simulink model "PMLSM_MIL_ControlCore_Sim"  (R2026a)
settings: Solver=FixedStepDiscrete  StopTime=MIL_StopTime_s  FixedStep=MIL_Ts_s
InitFcn:
  | init_PMLSM_control_params; init_PMLSM_plant_params; init_PMLSM_mil_test_params;
values from neighbouring files (symbols this model uses):
  Inverter_DeadTime_Mode = 0    [init_PMLSM_mil_test_params.m]
  MIL_Current_Control_Ts_s = 1e-4    (= 0.0001)    [init_PMLSM_mil_test_params.m]
  MIL_EnableTime_s = 0.1    [init_PMLSM_mil_test_params.m]
  MIL_Fault_Start_s = 2.0    (= 2)    [init_PMLSM_mil_test_params.m]
  MIL_Fault_Test_Case = 0    [init_PMLSM_mil_test_params.m]
  MIL_InitDoneDelay_s = 1    [init_PMLSM_mil_test_params.m]
  MIL_Mode = 1    [init_PMLSM_mil_test_params.m]
  MIL_PWM_Delay_Substep_s = MIL_Ts_s    (= 0.0001)    [init_PMLSM_mil_test_params.m]
  MIL_PWM_Update_Delay_Accurate_Enable = 0    [init_PMLSM_mil_test_params.m]
  MIL_PWM_Update_Delay_Mode = 1    [init_PMLSM_mil_test_params.m]
  MIL_StaticCurrentStepTest_Enable = 1    [init_PMLSM_mil_test_params.m]
  MIL_Ts_s = 1e-4    (= 0.0001)    [init_PMLSM_mil_test_params.m]
  Plant_Input_Mode = 2    [init_PMLSM_mil_test_params.m]
  PMLSM_Bv_N_per_mps = 0    [init_PMLSM_ThreeLoop_Simple.m]    (also in init_PMLSM_plant_params.m)
  PMLSM_deadtime_current_eps_A = 1e-4    (= 0.0001)    [init_PMLSM_ThreeLoop_Simple.m]    (also in init_PMLSM_plant_params.m)
  PMLSM_deadtime_ratio = PMLSM_deadtime_s/Ts    (= 0.01)    [init_PMLSM_ThreeLoop_Simple.m]    (also in init_PMLSM_plant_params.m)
  PMLSM_Fc_N = 0    [init_PMLSM_ThreeLoop_Simple.m]    (also in init_PMLSM_plant_params.m)
  PMLSM_grating_resolution_mm = 0.0001    [init_PMLSM_plant_params.m]
  PMLSM_Kf_peak_N_per_Apeak = 31.4/sqrt(2)    [init_PMLSM_ThreeLoop_Simple.m]    (also in init_PMLSM_plant_params.m = PMLSM_Kf_rms_N_per_Arms/sqrt(2))
  PMLSM_Ld_H = Ld    (= 0.001745)    [PMSLM_Init_Params_MBDL4.m]    (also in init_PMLSM_ThreeLoop_Simple.m; init_PMLSM_plant_params.m)
  PMLSM_Lq_H = Lq    (= 0.001745)    [PMSLM_Init_Params_MBDL4.m]    (also in init_PMLSM_ThreeLoop_Simple.m; init_PMLSM_plant_params.m)
  PMLSM_M_kg = 0.91    [init_PMLSM_ThreeLoop_Simple.m]    (also in init_PMLSM_plant_params.m)
  PMLSM_psi_f_Wb = flux    (= 0.141)    [PMSLM_Init_Params_MBDL4.m]    (also in init_PMLSM_ThreeLoop_Simple.m; init_PMLSM_plant_params.m)
  PMLSM_pwm_period_counts = CPU_Clock*Ts/2    (= 10000)    [init_PMLSM_ThreeLoop_Simple.m]    (also in init_PMLSM_plant_params.m = 7500)
  PMLSM_Rs_ohm = Rs    (= 2.37)    [PMSLM_Init_Params_MBDL4.m]    (also in init_PMLSM_ThreeLoop_Simple.m; init_PMLSM_plant_params.m)
  PMLSM_sensor_delay_samples = 50    [init_PMLSM_plant_params.m]
  PMLSM_tau_NN_m = 0.06    [init_PMLSM_ThreeLoop_Simple.m]    (also in init_PMLSM_plant_params.m)
  PMLSM_theta_offset_rad = 0    [init_PMLSM_ThreeLoop_Simple.m]    (also in init_PMLSM_plant_params.m)
  PMLSM_Ts_s = Ts/2    (= 5e-05)    [init_PMLSM_ThreeLoop_Simple.m]    (also in init_PMLSM_plant_params.m = 0.0001)
  PMLSM_v_eps_mps = 1e-3    (= 0.001)    [init_PMLSM_ThreeLoop_Simple.m]    (also in init_PMLSM_plant_params.m)
  Ts_ACR = 1e-4    (= 0.0001)    [PMSLM_Init_Params_MBDL4.m]    (also in init_PMLSM_ThreeLoop_Simple.m)
undefined symbols (not defined in the file or in its folder): DiscIntNeverNeededParam
settings Model: Creator=lww  LastModifiedBy=lww

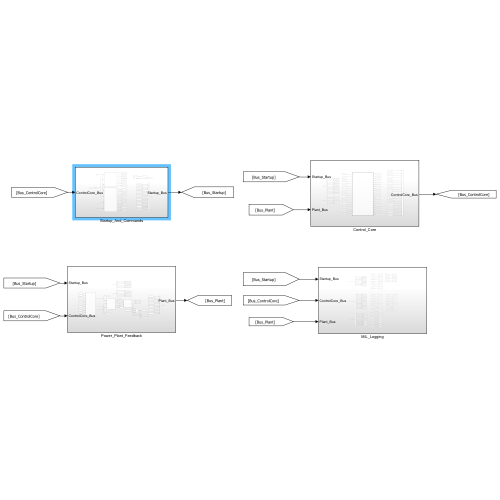
[thumbnail: Simulink's stored preview of the top-level diagram]
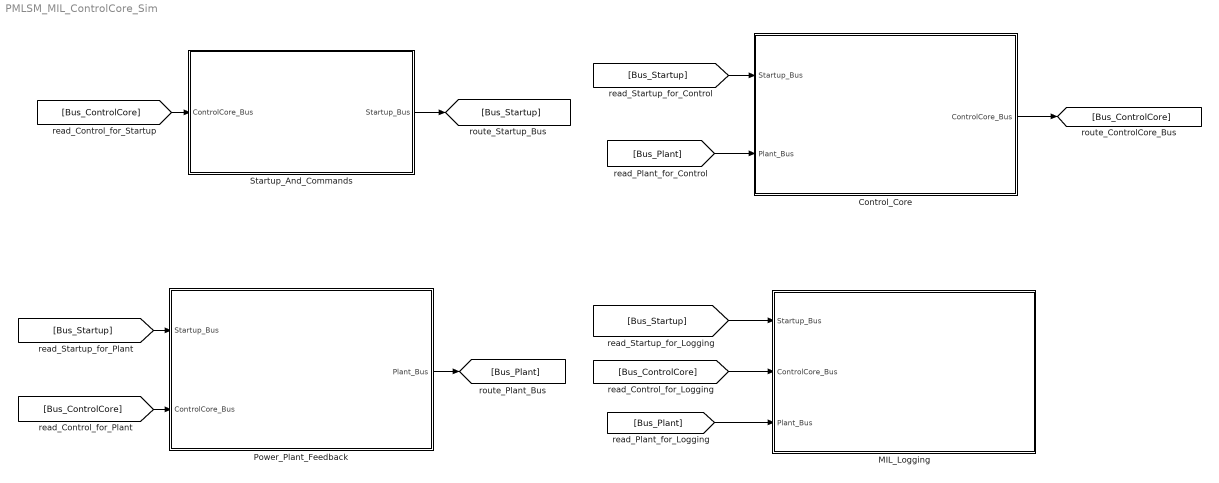
== system PMLSM_MIL_ControlCore_Sim ==
  Control_Core : Subsystem
  MIL_Logging : Subsystem
  Power_Plant_Feedback : Subsystem
  Startup_And_Commands : Subsystem
  wires:
  Startup_And_Commands/1(Startup_Bus) -> [Bus_Startup]
  [Bus_Startup] -> Control_Core/1(Startup_Bus)
  [Bus_Startup] -> Power_Plant_Feedback/1(Startup_Bus)
  [Bus_Startup] -> MIL_Logging/1(Startup_Bus)
  Control_Core/1(ControlCore_Bus) -> [Bus_ControlCore]
  [Bus_ControlCore] -> Startup_And_Commands/1(ControlCore_Bus)
  [Bus_ControlCore] -> Power_Plant_Feedback/2(ControlCore_Bus)
  [Bus_ControlCore] -> MIL_Logging/2(ControlCore_Bus)
  Power_Plant_Feedback/1(Plant_Bus) -> [Bus_Plant]
  [Bus_Plant] -> Control_Core/2(Plant_Bus)
  [Bus_Plant] -> MIL_Logging/3(Plant_Bus)

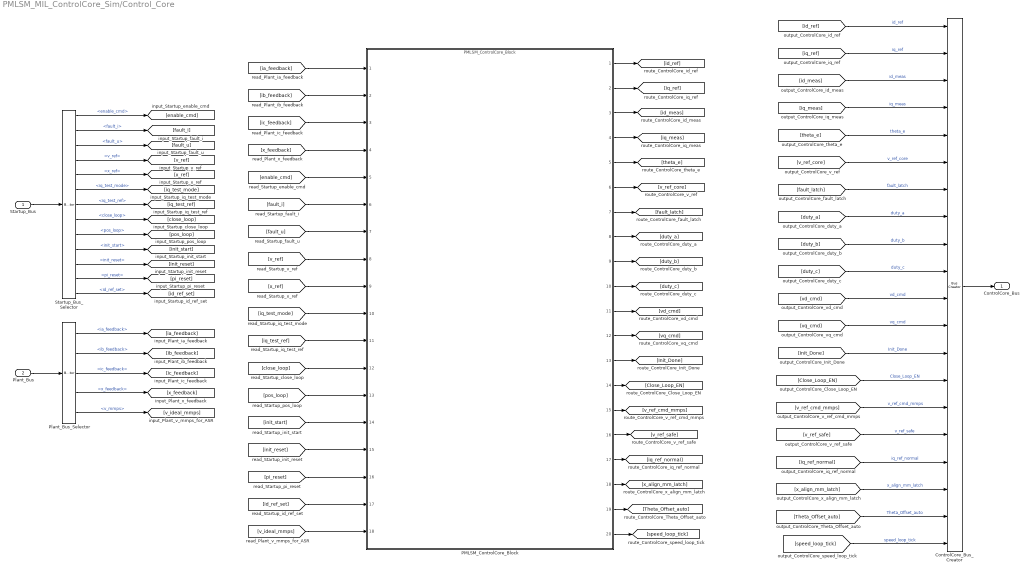
== system PMLSM_MIL_ControlCore_Sim/Control_Core ==
  Startup_Bus : Inport
  Plant_Bus : Inport  Port=2
  ControlCore_Bus_Creator : BusCreator  Inputs=20
  PMLSM_ControlCore_Block : ModelReference  ModelNameDialog=PMLSM_ControlCore_Block  SimulationMode=Normal  ModelReferenceVersion=6.250
  Plant_Bus_Selector : BusSelector  OutputSignals=ia_feedback,ib_feedback,ic_feedback,x_feedback,v_mmps
  Startup_Bus_Selector : BusSelector  OutputSignals=enable_cmd,fault_i,fault_u,v_ref,x_ref,iq_test_mode,iq_test_ref,close_loop,pos_loop,init_start,init_reset,pi_reset,id_ref_set
  ControlCore_Bus : Outport
  wires:
  Startup_Bus/1 -> Startup_Bus_Selector/1
  Startup_Bus_Selector/1 -> [enable_cmd]  "<enable_cmd>"
  Startup_Bus_Selector/2 -> [fault_i]  "<fault_i>"
  Startup_Bus_Selector/3 -> [fault_u]  "<fault_u>"
  Startup_Bus_Selector/4 -> [v_ref]  "<v_ref>"
  Startup_Bus_Selector/5 -> [x_ref]  "<x_ref>"
  Startup_Bus_Selector/6 -> [iq_test_mode]  "<iq_test_mode>"
  Startup_Bus_Selector/7 -> [iq_test_ref]  "<iq_test_ref>"
  Startup_Bus_Selector/8 -> [close_loop]  "<close_loop>"
  Startup_Bus_Selector/9 -> [pos_loop]  "<pos_loop>"
  Startup_Bus_Selector/10 -> [init_start]  "<init_start>"
  Startup_Bus_Selector/11 -> [init_reset]  "<init_reset>"
  Startup_Bus_Selector/12 -> [pi_reset]  "<pi_reset>"
  Startup_Bus_Selector/13 -> [id_ref_set]  "<id_ref_set>"
  Plant_Bus/1 -> Plant_Bus_Selector/1
  Plant_Bus_Selector/1 -> [ia_feedback]  "<ia_feedback>"
  Plant_Bus_Selector/2 -> [ib_feedback]  "<ib_feedback>"
  Plant_Bus_Selector/3 -> [ic_feedback]  "<ic_feedback>"
  Plant_Bus_Selector/4 -> [x_feedback]  "<x_feedback>"
  [ia_feedback] -> PMLSM_ControlCore_Block/1
  [ib_feedback] -> PMLSM_ControlCore_Block/2
  [ic_feedback] -> PMLSM_ControlCore_Block/3
  [x_feedback] -> PMLSM_ControlCore_Block/4
  [enable_cmd] -> PMLSM_ControlCore_Block/5
  [fault_i] -> PMLSM_ControlCore_Block/6
  [fault_u] -> PMLSM_ControlCore_Block/7
  [v_ref] -> PMLSM_ControlCore_Block/8
  [x_ref] -> PMLSM_ControlCore_Block/9
  [iq_test_mode] -> PMLSM_ControlCore_Block/10
  [iq_test_ref] -> PMLSM_ControlCore_Block/11
  [close_loop] -> PMLSM_ControlCore_Block/12
  [pos_loop] -> PMLSM_ControlCore_Block/13
  [init_start] -> PMLSM_ControlCore_Block/14
  [init_reset] -> PMLSM_ControlCore_Block/15
  [pi_reset] -> PMLSM_ControlCore_Block/16
  [id_ref_set] -> PMLSM_ControlCore_Block/17
  PMLSM_ControlCore_Block/1 -> [id_ref]
  PMLSM_ControlCore_Block/2 -> [iq_ref]
  PMLSM_ControlCore_Block/3 -> [id_meas]
  PMLSM_ControlCore_Block/4 -> [iq_meas]
  PMLSM_ControlCore_Block/5 -> [theta_e]
  PMLSM_ControlCore_Block/6 -> [v_ref_core]
  PMLSM_ControlCore_Block/7 -> [fault_latch]
  PMLSM_ControlCore_Block/8 -> [duty_a]
  PMLSM_ControlCore_Block/9 -> [duty_b]
  PMLSM_ControlCore_Block/10 -> [duty_c]
  PMLSM_ControlCore_Block/11 -> [vd_cmd]
  PMLSM_ControlCore_Block/12 -> [vq_cmd]
  PMLSM_ControlCore_Block/13 -> [Init_Done]
  PMLSM_ControlCore_Block/14 -> [Close_Loop_EN]
  PMLSM_ControlCore_Block/15 -> [v_ref_cmd_mmps]
  PMLSM_ControlCore_Block/16 -> [v_ref_safe]
  PMLSM_ControlCore_Block/17 -> [iq_ref_normal]
  PMLSM_ControlCore_Block/18 -> [x_align_mm_latch]
  PMLSM_ControlCore_Block/19 -> [Theta_Offset_auto]
  [id_ref] -> ControlCore_Bus_Creator/1  "id_ref"
  [iq_ref] -> ControlCore_Bus_Creator/2  "iq_ref"
  [id_meas] -> ControlCore_Bus_Creator/3  "id_meas"
  [iq_meas] -> ControlCore_Bus_Creator/4  "iq_meas"
  [theta_e] -> ControlCore_Bus_Creator/5  "theta_e"
  [v_ref_core] -> ControlCore_Bus_Creator/6  "v_ref_core"
  [fault_latch] -> ControlCore_Bus_Creator/7  "fault_latch"
  [duty_a] -> ControlCore_Bus_Creator/8  "duty_a"
  [duty_b] -> ControlCore_Bus_Creator/9  "duty_b"
  [duty_c] -> ControlCore_Bus_Creator/10  "duty_c"
  [vd_cmd] -> ControlCore_Bus_Creator/11  "vd_cmd"
  [vq_cmd] -> ControlCore_Bus_Creator/12  "vq_cmd"
  [Init_Done] -> ControlCore_Bus_Creator/13  "Init_Done"
  [Close_Loop_EN] -> ControlCore_Bus_Creator/14  "Close_Loop_EN"
  [v_ref_cmd_mmps] -> ControlCore_Bus_Creator/15  "v_ref_cmd_mmps"
  [v_ref_safe] -> ControlCore_Bus_Creator/16  "v_ref_safe"
  [iq_ref_normal] -> ControlCore_Bus_Creator/17  "iq_ref_normal"
  [x_align_mm_latch] -> ControlCore_Bus_Creator/18  "x_align_mm_latch"
  [Theta_Offset_auto] -> ControlCore_Bus_Creator/19  "Theta_Offset_auto"
  ControlCore_Bus_Creator/1 -> ControlCore_Bus/1
  Plant_Bus_Selector/5 -> [v_ideal_mmps]  "<v_mmps>"
  [v_ideal_mmps] -> PMLSM_ControlCore_Block/18
  PMLSM_ControlCore_Block/20 -> [speed_loop_tick]
  [speed_loop_tick] -> ControlCore_Bus_Creator/20  "speed_loop_tick"

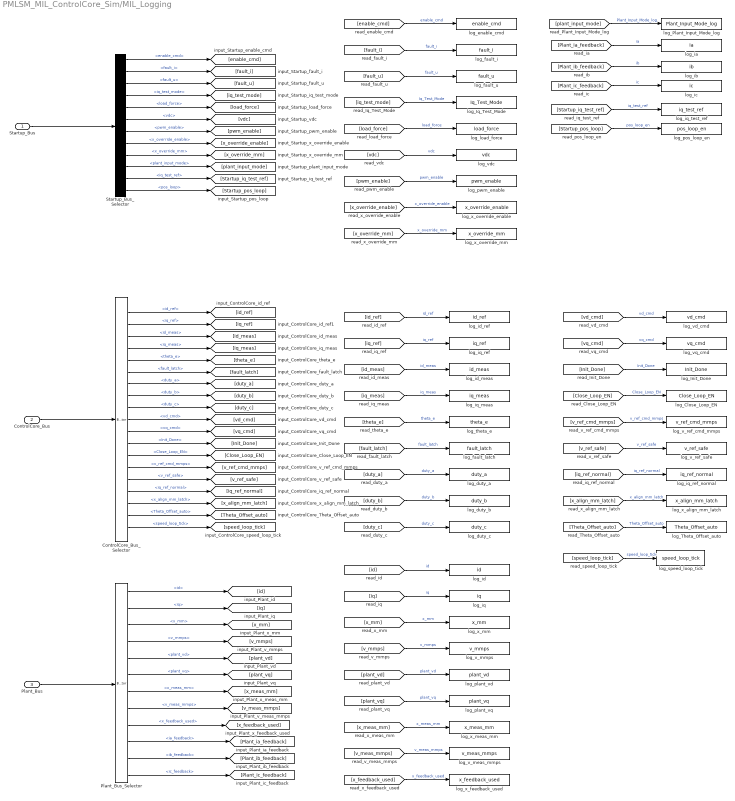
== system PMLSM_MIL_ControlCore_Sim/MIL_Logging ==
  Startup_Bus : Inport
  ControlCore_Bus : Inport  Port=2
  Plant_Bus : Inport  Port=3
  ControlCore_Bus_Selector : BusSelector  OutputSignals=id_ref,iq_ref,id_meas,iq_meas,theta_e,fault_latch,duty_a,duty_b,duty_c,vd_cmd,vq_cmd,Init_Done,Close_Loop_EN,v_ref_cmd_mmps,v_ref_safe,iq_ref_normal,x_align_mm_latch,Theta_Offset_auto,speed_loop_tick
  Plant_Bus_Selector : BusSelector  OutputSignals=id,iq,x_mm,v_mmps,plant_vd,plant_vq,x_meas_mm,v_meas_mmps,x_feedback_used,ia_feedback,ib_feedback,ic_feedback
  Startup_Bus_Selector : BusSelector  OutputSignals=enable_cmd,fault_i,fault_u,iq_test_mode,load_force,vdc,pwm_enable,x_override_enable,x_override_mm,plant_input_mode,iq_test_ref,pos_loop
  log_Close_Loop_EN : ToWorkspace  VariableName=Close_Loop_EN  SaveFormat=Timeseries  SampleTime=-1
  log_Init_Done : ToWorkspace  VariableName=Init_Done  SaveFormat=Timeseries  SampleTime=-1
  log_Iq_Test_Mode : ToWorkspace  VariableName=Iq_Test_Mode  SaveFormat=Timeseries  SampleTime=-1
  log_Plant_Input_Mode_log : ToWorkspace  VariableName=Plant_Input_Mode_log  SaveFormat=Timeseries  SampleTime=-1
  log_Theta_Offset_auto : ToWorkspace  VariableName=Theta_Offset_auto  SaveFormat=Timeseries  SampleTime=-1
  log_duty_a : ToWorkspace  VariableName=duty_a  SaveFormat=Timeseries  SampleTime=-1
  log_duty_b : ToWorkspace  VariableName=duty_b  SaveFormat=Timeseries  SampleTime=-1
  log_duty_c : ToWorkspace  VariableName=duty_c  SaveFormat=Timeseries  SampleTime=-1
  log_enable_cmd : ToWorkspace  VariableName=enable_cmd  SaveFormat=Timeseries  SampleTime=-1
  log_fault_i : ToWorkspace  VariableName=fault_i  SaveFormat=Timeseries  SampleTime=-1
  log_fault_latch : ToWorkspace  VariableName=fault_latch  SaveFormat=Timeseries  SampleTime=-1
  log_fault_u : ToWorkspace  VariableName=fault_u  SaveFormat=Timeseries  SampleTime=-1
  log_ia : ToWorkspace  VariableName=ia  SaveFormat=Timeseries  SampleTime=-1
  log_ib : ToWorkspace  VariableName=ib  SaveFormat=Timeseries  SampleTime=-1
  log_ic : ToWorkspace  VariableName=ic  SaveFormat=Timeseries  SampleTime=-1
  log_id : ToWorkspace  VariableName=id  SaveFormat=Timeseries  SampleTime=-1
  log_id_meas : ToWorkspace  VariableName=id_meas  SaveFormat=Timeseries  SampleTime=-1
  log_id_ref : ToWorkspace  VariableName=id_ref  SaveFormat=Timeseries  SampleTime=-1
  log_iq : ToWorkspace  VariableName=iq  SaveFormat=Timeseries  SampleTime=-1
  log_iq_meas : ToWorkspace  VariableName=iq_meas  SaveFormat=Timeseries  SampleTime=-1
  log_iq_ref : ToWorkspace  VariableName=iq_ref  SaveFormat=Timeseries  SampleTime=-1
  log_iq_ref_normal : ToWorkspace  VariableName=iq_ref_normal  SaveFormat=Timeseries  SampleTime=-1
  log_iq_test_ref : ToWorkspace  VariableName=iq_test_ref  SaveFormat=Timeseries  SampleTime=-1
  log_load_force : ToWorkspace  VariableName=load_force  SaveFormat=Timeseries  SampleTime=-1
  log_plant_vd : ToWorkspace  VariableName=plant_vd  SaveFormat=Timeseries  SampleTime=-1
  log_plant_vq : ToWorkspace  VariableName=plant_vq  SaveFormat=Timeseries  SampleTime=-1
  log_pos_loop_en : ToWorkspace  VariableName=pos_loop_en  SaveFormat=Timeseries  SampleTime=-1
  log_pwm_enable : ToWorkspace  VariableName=pwm_enable  SaveFormat=Timeseries  SampleTime=-1
  log_speed_loop_tick : ToWorkspace  VariableName=speed_loop_tick  SaveFormat=Structure With Time  SampleTime=-1
  log_theta_e : ToWorkspace  VariableName=theta_e  SaveFormat=Timeseries  SampleTime=-1
  log_v_meas_mmps : ToWorkspace  VariableName=v_meas_mmps  SaveFormat=Timeseries  SampleTime=-1
  log_v_mmps : ToWorkspace  VariableName=v_mmps  SaveFormat=Timeseries  SampleTime=-1
  log_v_ref_cmd_mmps : ToWorkspace  VariableName=v_ref_cmd_mmps  SaveFormat=Timeseries  SampleTime=-1
  log_v_ref_safe : ToWorkspace  VariableName=v_ref_safe  SaveFormat=Timeseries  SampleTime=-1
  log_vd_cmd : ToWorkspace  VariableName=vd_cmd  SaveFormat=Timeseries  SampleTime=-1
  log_vdc : ToWorkspace  VariableName=vdc  SaveFormat=Timeseries  SampleTime=-1
  log_vq_cmd : ToWorkspace  VariableName=vq_cmd  SaveFormat=Timeseries  SampleTime=-1
  log_x_align_mm_latch : ToWorkspace  VariableName=x_align_mm_latch  SaveFormat=Timeseries  SampleTime=-1
  log_x_feedback_used : ToWorkspace  VariableName=x_feedback_used  SaveFormat=Timeseries  SampleTime=-1
  log_x_meas_mm : ToWorkspace  VariableName=x_meas_mm  SaveFormat=Timeseries  SampleTime=-1
  log_x_mm : ToWorkspace  VariableName=x_mm  SaveFormat=Timeseries  SampleTime=-1
  log_x_override_enable : ToWorkspace  VariableName=x_override_enable  SaveFormat=Timeseries  SampleTime=-1
  log_x_override_mm : ToWorkspace  VariableName=x_override_mm  SaveFormat=Timeseries  SampleTime=-1
  wires:
  Startup_Bus/1 -> Startup_Bus_Selector/1
  Startup_Bus_Selector/1 -> [enable_cmd]  "<enable_cmd>"
  Startup_Bus_Selector/2 -> [fault_i]  "<fault_i>"
  Startup_Bus_Selector/3 -> [fault_u]  "<fault_u>"
  Startup_Bus_Selector/4 -> [iq_test_mode]  "<iq_test_mode>"
  Startup_Bus_Selector/5 -> [load_force]  "<load_force>"
  Startup_Bus_Selector/6 -> [vdc]  "<vdc>"
  Startup_Bus_Selector/7 -> [pwm_enable]  "<pwm_enable>"
  Startup_Bus_Selector/8 -> [x_override_enable]  "<x_override_enable>"
  Startup_Bus_Selector/9 -> [x_override_mm]  "<x_override_mm>"
  Startup_Bus_Selector/10 -> [plant_input_mode]  "<plant_input_mode>"
  ControlCore_Bus/1 -> ControlCore_Bus_Selector/1
  ControlCore_Bus_Selector/1 -> [id_ref]  "<id_ref>"
  ControlCore_Bus_Selector/2 -> [iq_ref]  "<iq_ref>"
  ControlCore_Bus_Selector/3 -> [id_meas]  "<id_meas>"
  ControlCore_Bus_Selector/4 -> [iq_meas]  "<iq_meas>"
  ControlCore_Bus_Selector/5 -> [theta_e]  "<theta_e>"
  ControlCore_Bus_Selector/6 -> [fault_latch]  "<fault_latch>"
  ControlCore_Bus_Selector/7 -> [duty_a]  "<duty_a>"
  ControlCore_Bus_Selector/8 -> [duty_b]  "<duty_b>"
  ControlCore_Bus_Selector/9 -> [duty_c]  "<duty_c>"
  ControlCore_Bus_Selector/10 -> [vd_cmd]  "<vd_cmd>"
  ControlCore_Bus_Selector/11 -> [vq_cmd]  "<vq_cmd>"
  ControlCore_Bus_Selector/12 -> [Init_Done]  "<Init_Done>"
  ControlCore_Bus_Selector/13 -> [Close_Loop_EN]  "<Close_Loop_EN>"
  ControlCore_Bus_Selector/14 -> [v_ref_cmd_mmps]  "<v_ref_cmd_mmps>"
  ControlCore_Bus_Selector/15 -> [v_ref_safe]  "<v_ref_safe>"
  ControlCore_Bus_Selector/16 -> [iq_ref_normal]  "<iq_ref_normal>"
  ControlCore_Bus_Selector/17 -> [x_align_mm_latch]  "<x_align_mm_latch>"
  ControlCore_Bus_Selector/18 -> [Theta_Offset_auto]  "<Theta_Offset_auto>"
  Plant_Bus/1 -> Plant_Bus_Selector/1
  Plant_Bus_Selector/1 -> [id]  "<id>"
  Plant_Bus_Selector/2 -> [iq]  "<iq>"
  Plant_Bus_Selector/3 -> [x_mm]  "<x_mm>"
  Plant_Bus_Selector/4 -> [v_mmps]  "<v_mmps>"
  Plant_Bus_Selector/5 -> [plant_vd]  "<plant_vd>"
  Plant_Bus_Selector/6 -> [plant_vq]  "<plant_vq>"
  Plant_Bus_Selector/7 -> [x_meas_mm]  "<x_meas_mm>"
  Plant_Bus_Selector/8 -> [v_meas_mmps]  "<v_meas_mmps>"
  Plant_Bus_Selector/9 -> [x_feedback_used]  "<x_feedback_used>"
  [id] -> log_id/1  "id"
  [iq] -> log_iq/1  "iq"
  [x_mm] -> log_x_mm/1  "x_mm"
  [v_mmps] -> log_v_mmps/1  "v_mmps"
  [plant_vd] -> log_plant_vd/1  "plant_vd"
  [plant_vq] -> log_plant_vq/1  "plant_vq"
  [x_meas_mm] -> log_x_meas_mm/1  "x_meas_mm"
  [v_meas_mmps] -> log_v_meas_mmps/1  "v_meas_mmps"
  [x_feedback_used] -> log_x_feedback_used/1  "x_feedback_used"
  [id_ref] -> log_id_ref/1  "id_ref"
  [iq_ref] -> log_iq_ref/1  "iq_ref"
  [id_meas] -> log_id_meas/1  "id_meas"
  [iq_meas] -> log_iq_meas/1  "iq_meas"
  [theta_e] -> log_theta_e/1  "theta_e"
  [fault_latch] -> log_fault_latch/1  "fault_latch"
  [duty_a] -> log_duty_a/1  "duty_a"
  [duty_b] -> log_duty_b/1  "duty_b"
  [duty_c] -> log_duty_c/1  "duty_c"
  [vd_cmd] -> log_vd_cmd/1  "vd_cmd"
  [vq_cmd] -> log_vq_cmd/1  "vq_cmd"
  [Init_Done] -> log_Init_Done/1  "Init_Done"
  [Close_Loop_EN] -> log_Close_Loop_EN/1  "Close_Loop_EN"
  [v_ref_cmd_mmps] -> log_v_ref_cmd_mmps/1  "v_ref_cmd_mmps"
  [v_ref_safe] -> log_v_ref_safe/1  "v_ref_safe"
  [iq_ref_normal] -> log_iq_ref_normal/1  "iq_ref_normal"
  [x_align_mm_latch] -> log_x_align_mm_latch/1  "x_align_mm_latch"
  [Theta_Offset_auto] -> log_Theta_Offset_auto/1  "Theta_Offset_auto"
  [enable_cmd] -> log_enable_cmd/1  "enable_cmd"
  [fault_i] -> log_fault_i/1  "fault_i"
  [fault_u] -> log_fault_u/1  "fault_u"
  [iq_test_mode] -> log_Iq_Test_Mode/1  "Iq_Test_Mode"
  [load_force] -> log_load_force/1  "load_force"
  [vdc] -> log_vdc/1  "vdc"
  [pwm_enable] -> log_pwm_enable/1  "pwm_enable"
  [x_override_enable] -> log_x_override_enable/1  "x_override_enable"
  [x_override_mm] -> log_x_override_mm/1  "x_override_mm"
  [plant_input_mode] -> log_Plant_Input_Mode_log/1  "Plant_Input_Mode_log"
  Startup_Bus_Selector/11 -> [Startup_iq_test_ref]  "<iq_test_ref>"
  Startup_Bus_Selector/12 -> [Startup_pos_loop]  "<pos_loop>"
  Plant_Bus_Selector/10 -> [Plant_ia_feedback]  "<ia_feedback>"
  Plant_Bus_Selector/11 -> [Plant_ib_feedback]  "<ib_feedback>"
  Plant_Bus_Selector/12 -> [Plant_ic_feedback]  "<ic_feedback>"
  [Startup_iq_test_ref] -> log_iq_test_ref/1  "iq_test_ref"
  [Startup_pos_loop] -> log_pos_loop_en/1  "pos_loop_en"
  [Plant_ia_feedback] -> log_ia/1  "ia"
  [Plant_ib_feedback] -> log_ib/1  "ib"
  [Plant_ic_feedback] -> log_ic/1  "ic"
  [speed_loop_tick] -> log_speed_loop_tick/1  "speed_loop_tick"
  ControlCore_Bus_Selector/19 -> [speed_loop_tick]  "<speed_loop_tick>"

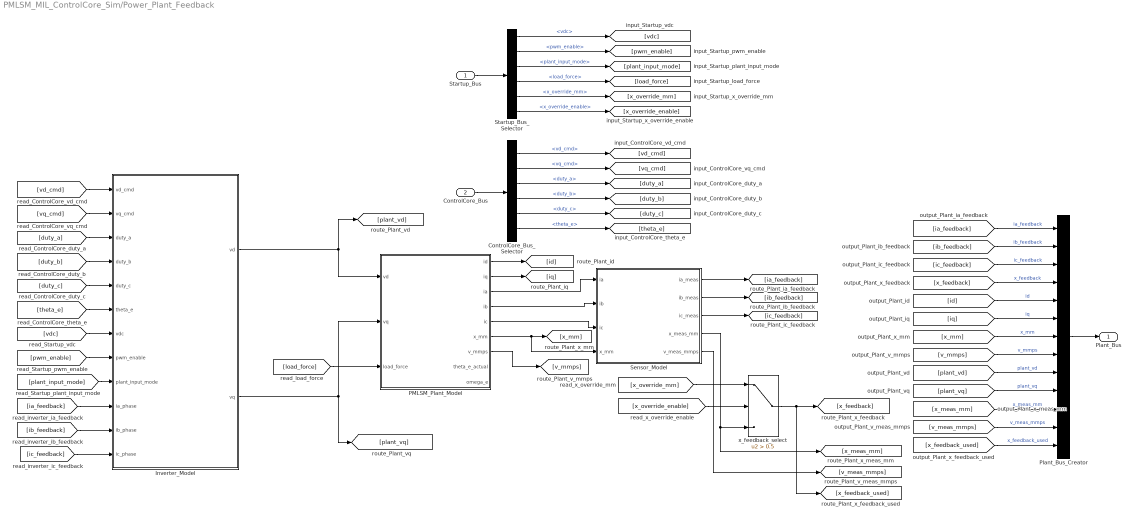
== system PMLSM_MIL_ControlCore_Sim/Power_Plant_Feedback ==
  Startup_Bus : Inport
  ControlCore_Bus : Inport  Port=2
  ControlCore_Bus_Selector : BusSelector  OutputSignals=vd_cmd,vq_cmd,duty_a,duty_b,duty_c,theta_e
  Inverter_Model : Subsystem
  PMLSM_Plant_Model : Subsystem
  Plant_Bus_Creator : BusCreator  Inputs=13
  Sensor_Model : Subsystem
  Startup_Bus_Selector : BusSelector  OutputSignals=vdc,pwm_enable,plant_input_mode,load_force,x_override_mm,x_override_enable
  x_feedback_select : Switch  Criteria=u2 > Threshold  Threshold=0.5  SaturateOnIntegerOverflow=off  InputSameDT=off
  Plant_Bus : Outport
  wires:
  Startup_Bus/1 -> Startup_Bus_Selector/1
  Startup_Bus_Selector/1 -> [vdc]  "<vdc>"
  Startup_Bus_Selector/2 -> [pwm_enable]  "<pwm_enable>"
  Startup_Bus_Selector/3 -> [plant_input_mode]  "<plant_input_mode>"
  Startup_Bus_Selector/4 -> [load_force]  "<load_force>"
  Startup_Bus_Selector/5 -> [x_override_mm]  "<x_override_mm>"
  Startup_Bus_Selector/6 -> [x_override_enable]  "<x_override_enable>"
  ControlCore_Bus/1 -> ControlCore_Bus_Selector/1
  ControlCore_Bus_Selector/1 -> [vd_cmd]  "<vd_cmd>"
  ControlCore_Bus_Selector/2 -> [vq_cmd]  "<vq_cmd>"
  ControlCore_Bus_Selector/3 -> [duty_a]  "<duty_a>"
  ControlCore_Bus_Selector/4 -> [duty_b]  "<duty_b>"
  ControlCore_Bus_Selector/5 -> [duty_c]  "<duty_c>"
  ControlCore_Bus_Selector/6 -> [theta_e]  "<theta_e>"
  [vd_cmd] -> Inverter_Model/1(vd_cmd)
  [vq_cmd] -> Inverter_Model/2(vq_cmd)
  [duty_a] -> Inverter_Model/3(duty_a)
  [duty_b] -> Inverter_Model/4(duty_b)
  [duty_c] -> Inverter_Model/5(duty_c)
  [theta_e] -> Inverter_Model/6(theta_e)
  [vdc] -> Inverter_Model/7(vdc)
  [pwm_enable] -> Inverter_Model/8(pwm_enable)
  [plant_input_mode] -> Inverter_Model/9(plant_input_mode)
  [load_force] -> PMLSM_Plant_Model/3(load_force)
  Inverter_Model/1(vd) -> [plant_vd], PMLSM_Plant_Model/1(vd)
  Inverter_Model/2(vq) -> PMLSM_Plant_Model/2(vq), [plant_vq]
  PMLSM_Plant_Model/3(ia) -> Sensor_Model/1(ia)
  PMLSM_Plant_Model/4(ib) -> Sensor_Model/2(ib)
  PMLSM_Plant_Model/6(x_mm) -> Sensor_Model/4(x_mm), [x_mm]
  Sensor_Model/1(ia_meas) -> [ia_feedback]
  Sensor_Model/2(ib_meas) -> [ib_feedback]
  [x_override_mm] -> x_feedback_select/1
  [x_override_enable] -> x_feedback_select/2
  Sensor_Model/4(x_meas_mm) -> [x_meas_mm], x_feedback_select/3
  x_feedback_select/1 -> [x_feedback_used], [x_feedback]
  PMLSM_Plant_Model/1(id) -> [id]
  PMLSM_Plant_Model/2(iq) -> [iq]
  PMLSM_Plant_Model/7(v_mmps) -> [v_mmps]
  [ia_feedback] -> Plant_Bus_Creator/1  "ia_feedback"
  [ib_feedback] -> Plant_Bus_Creator/2  "ib_feedback"
  [ic_feedback] -> Plant_Bus_Creator/3  "ic_feedback"
  [x_feedback] -> Plant_Bus_Creator/4  "x_feedback"
  [id] -> Plant_Bus_Creator/5  "id"
  [iq] -> Plant_Bus_Creator/6  "iq"
  [x_mm] -> Plant_Bus_Creator/7  "x_mm"
  [v_mmps] -> Plant_Bus_Creator/8  "v_mmps"
  [plant_vd] -> Plant_Bus_Creator/9  "plant_vd"
  [plant_vq] -> Plant_Bus_Creator/10  "plant_vq"
  [x_meas_mm] -> Plant_Bus_Creator/11  "x_meas_mm"
  [v_meas_mmps] -> Plant_Bus_Creator/12  "v_meas_mmps"
  [x_feedback_used] -> Plant_Bus_Creator/13  "x_feedback_used"
  Plant_Bus_Creator/1 -> Plant_Bus/1
  Sensor_Model/3(ic_meas) -> [ic_feedback]
  Sensor_Model/5(v_meas_mmps) -> [v_meas_mmps]
  PMLSM_Plant_Model/5(ic) -> Sensor_Model/3(ic)
  [ia_feedback] -> Inverter_Model/10(ia_phase)
  [ib_feedback] -> Inverter_Model/11(ib_phase)
  [ic_feedback] -> Inverter_Model/12(ic_phase)

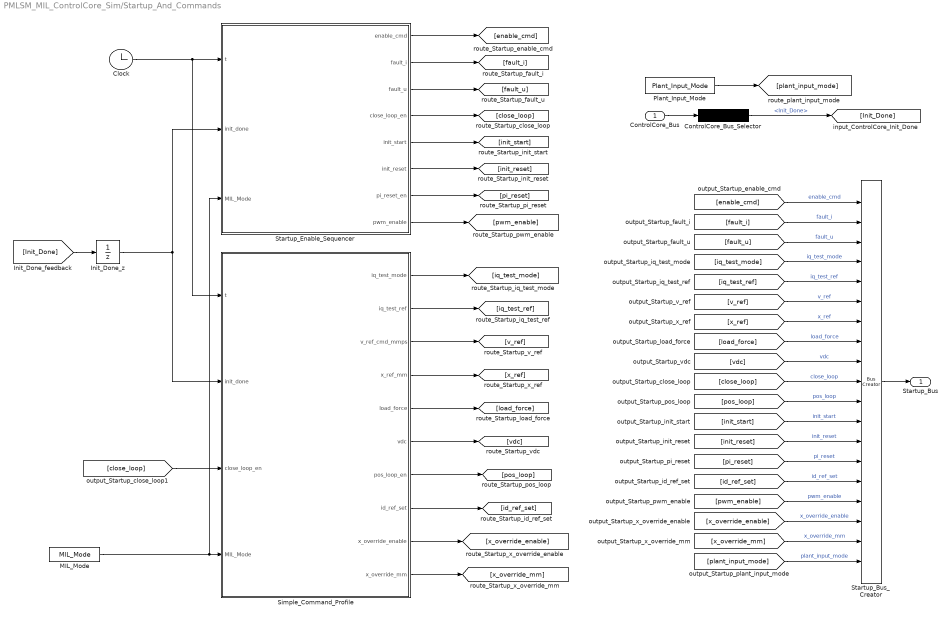
== system PMLSM_MIL_ControlCore_Sim/Startup_And_Commands ==
  ControlCore_Bus : Inport
  Clock : Clock
  ControlCore_Bus_Selector : BusSelector  OutputSignals=Init_Done
  Init_Done_z : UnitDelay  SampleTime=1e-4
  MIL_Mode : Constant  Value=MIL_Mode
  Plant_Input_Mode : Constant  Value=Plant_Input_Mode
  Simple_Command_Profile : MATLAB Function  TreatAsAtomicUnit=on
  Startup_Bus_Creator : BusCreator  Inputs=19
  Startup_Enable_Sequencer : MATLAB Function  TreatAsAtomicUnit=on
  Startup_Bus : Outport
  wires:
  ControlCore_Bus/1 -> ControlCore_Bus_Selector/1
  ControlCore_Bus_Selector/1 -> [Init_Done]  "<Init_Done>"
  [Init_Done] -> Init_Done_z/1
  Init_Done_z/1 -> Simple_Command_Profile/2(init_done), Startup_Enable_Sequencer/2(init_done)
  Plant_Input_Mode/1 -> [plant_input_mode]
  [enable_cmd] -> Startup_Bus_Creator/1  "enable_cmd"
  [fault_i] -> Startup_Bus_Creator/2  "fault_i"
  [fault_u] -> Startup_Bus_Creator/3  "fault_u"
  [iq_test_mode] -> Startup_Bus_Creator/4  "iq_test_mode"
  [iq_test_ref] -> Startup_Bus_Creator/5  "iq_test_ref"
  [v_ref] -> Startup_Bus_Creator/6  "v_ref"
  [x_ref] -> Startup_Bus_Creator/7  "x_ref"
  [load_force] -> Startup_Bus_Creator/8  "load_force"
  [vdc] -> Startup_Bus_Creator/9  "vdc"
  [close_loop] -> Startup_Bus_Creator/10  "close_loop"
  [pos_loop] -> Startup_Bus_Creator/11  "pos_loop"
  [init_start] -> Startup_Bus_Creator/12  "init_start"
  [init_reset] -> Startup_Bus_Creator/13  "init_reset"
  [pi_reset] -> Startup_Bus_Creator/14  "pi_reset"
  [id_ref_set] -> Startup_Bus_Creator/15  "id_ref_set"
  [pwm_enable] -> Startup_Bus_Creator/16  "pwm_enable"
  [x_override_enable] -> Startup_Bus_Creator/17  "x_override_enable"
  [x_override_mm] -> Startup_Bus_Creator/18  "x_override_mm"
  [plant_input_mode] -> Startup_Bus_Creator/19  "plant_input_mode"
  Startup_Bus_Creator/1 -> Startup_Bus/1
  Clock/1 -> Simple_Command_Profile/1(t), Startup_Enable_Sequencer/1(t)
  Startup_Enable_Sequencer/4(close_loop_en) -> [close_loop]
  Startup_Enable_Sequencer/1(enable_cmd) -> [enable_cmd]
  Startup_Enable_Sequencer/2(fault_i) -> [fault_i]
  Startup_Enable_Sequencer/3(fault_u) -> [fault_u]
  Startup_Enable_Sequencer/5(init_start) -> [init_start]
  Startup_Enable_Sequencer/6(init_reset) -> [init_reset]
  Startup_Enable_Sequencer/7(pi_reset_en) -> [pi_reset]
  Startup_Enable_Sequencer/8(pwm_enable) -> [pwm_enable]
  Simple_Command_Profile/1(iq_test_mode) -> [iq_test_mode]
  Simple_Command_Profile/2(iq_test_ref) -> [iq_test_ref]
  Simple_Command_Profile/3(v_ref_cmd_mmps) -> [v_ref]
  Simple_Command_Profile/4(x_ref_mm) -> [x_ref]
  Simple_Command_Profile/5(load_force) -> [load_force]
  Simple_Command_Profile/6(vdc) -> [vdc]
  Simple_Command_Profile/7(pos_loop_en) -> [pos_loop]
  Simple_Command_Profile/8(id_ref_set) -> [id_ref_set]
  Simple_Command_Profile/9(x_override_enable) -> [x_override_enable]
  Simple_Command_Profile/10(x_override_mm) -> [x_override_mm]
  MIL_Mode/1 -> Startup_Enable_Sequencer/3(MIL_Mode), Simple_Command_Profile/4(MIL_Mode)
  [close_loop] -> Simple_Command_Profile/3(close_loop_en)

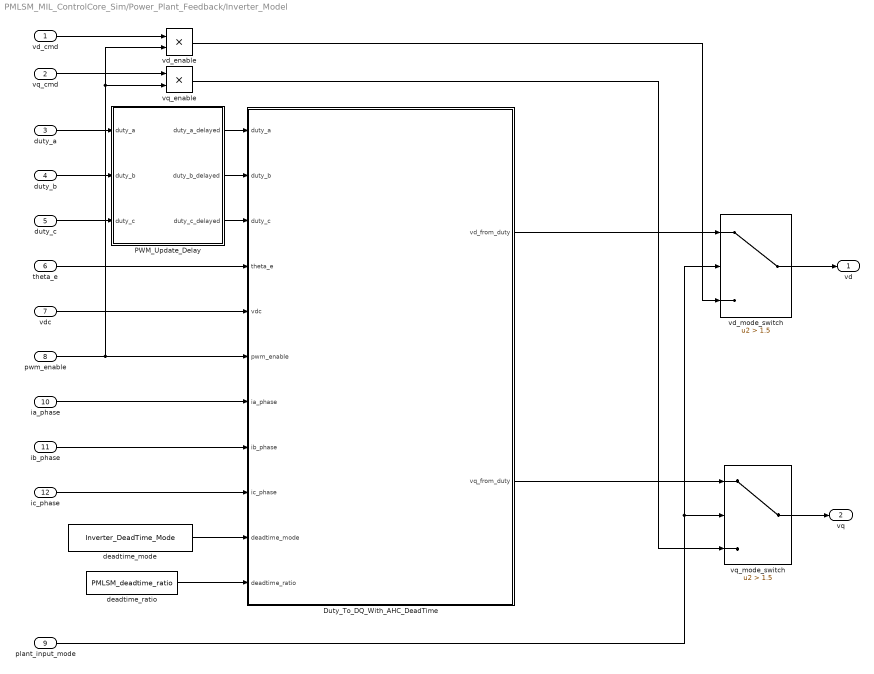
== system PMLSM_MIL_ControlCore_Sim/Power_Plant_Feedback/Inverter_Model ==
  vd_cmd : Inport
  vq_cmd : Inport  Port=2
  duty_a : Inport  Port=3
  duty_b : Inport  Port=4
  duty_c : Inport  Port=5
  theta_e : Inport  Port=6
  vdc : Inport  Port=7
  pwm_enable : Inport  Port=8
  plant_input_mode : Inport  Port=9
  ia_phase : Inport  Port=10
  ib_phase : Inport  Port=11
  ic_phase : Inport  Port=12
  Duty_To_DQ_With_AHC_DeadTime : Subsystem
  PWM_Update_Delay : Subsystem
  deadtime_mode : Constant  Value=Inverter_DeadTime_Mode
  deadtime_ratio : Constant  Value=PMLSM_deadtime_ratio
  vd_enable : Product
  vd_mode_switch : Switch  Criteria=u2 > Threshold  Threshold=1.5  SaturateOnIntegerOverflow=off  InputSameDT=off
  vq_enable : Product
  vq_mode_switch : Switch  Criteria=u2 > Threshold  Threshold=1.5  SaturateOnIntegerOverflow=off  InputSameDT=off
  vd : Outport
  vq : Outport  Port=2
  wires:
  vd_cmd/1 -> vd_enable/1
  pwm_enable/1 -> vd_enable/2, vq_enable/2, Duty_To_DQ_With_AHC_DeadTime/6(pwm_enable)
  vq_cmd/1 -> vq_enable/1
  theta_e/1 -> Duty_To_DQ_With_AHC_DeadTime/4(theta_e)
  vdc/1 -> Duty_To_DQ_With_AHC_DeadTime/5(vdc)
  ia_phase/1 -> Duty_To_DQ_With_AHC_DeadTime/7(ia_phase)
  ib_phase/1 -> Duty_To_DQ_With_AHC_DeadTime/8(ib_phase)
  ic_phase/1 -> Duty_To_DQ_With_AHC_DeadTime/9(ic_phase)
  deadtime_mode/1 -> Duty_To_DQ_With_AHC_DeadTime/10(deadtime_mode)
  deadtime_ratio/1 -> Duty_To_DQ_With_AHC_DeadTime/11(deadtime_ratio)
  Duty_To_DQ_With_AHC_DeadTime/1(vd_from_duty) -> vd_mode_switch/1
  plant_input_mode/1 -> vd_mode_switch/2, vq_mode_switch/2
  vd_enable/1 -> vd_mode_switch/3
  Duty_To_DQ_With_AHC_DeadTime/2(vq_from_duty) -> vq_mode_switch/1
  vq_enable/1 -> vq_mode_switch/3
  vd_mode_switch/1 -> vd/1
  vq_mode_switch/1 -> vq/1
  duty_a/1 -> PWM_Update_Delay/1(duty_a)
  duty_b/1 -> PWM_Update_Delay/2(duty_b)
  duty_c/1 -> PWM_Update_Delay/3(duty_c)
  PWM_Update_Delay/1(duty_a_delayed) -> Duty_To_DQ_With_AHC_DeadTime/1(duty_a)
  PWM_Update_Delay/2(duty_b_delayed) -> Duty_To_DQ_With_AHC_DeadTime/2(duty_b)
  PWM_Update_Delay/3(duty_c_delayed) -> Duty_To_DQ_With_AHC_DeadTime/3(duty_c)

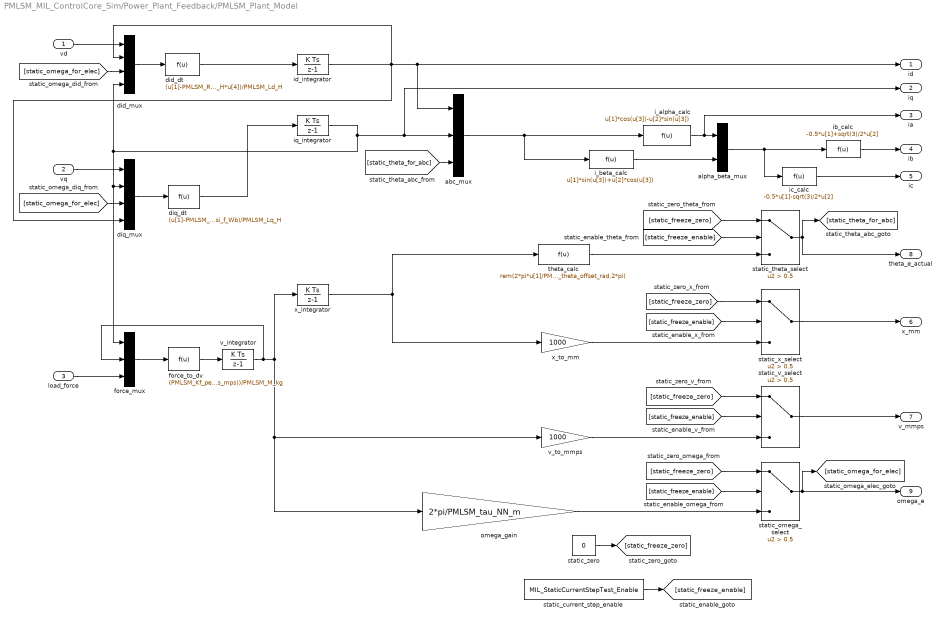
== system PMLSM_MIL_ControlCore_Sim/Power_Plant_Feedback/PMLSM_Plant_Model ==
  vd : Inport
  vq : Inport  Port=2
  load_force : Inport  Port=3
  abc_mux : Mux  Inputs=3
  alpha_beta_mux : Mux  Inputs=2
  did_dt : Fcn  Expr=(u[1]-PMLSM_Rs_ohm*u[2]+u[3]*PMLSM_Lq_H*u[4])/PMLSM_Ld_H
  did_mux : Mux
  diq_dt : Fcn  Expr=(u[1]-PMLSM_Rs_ohm*u[2]-u[3]*PMLSM_Ld_H*u[4]-u[3]*PMLSM_psi_f_Wb)/PMLSM_Lq_H
  diq_mux : Mux
  force_mux : Mux  Inputs=3
  force_to_dv : Fcn  Expr=(PMLSM_Kf_peak_N_per_Apeak*u[1]-u[3]-PMLSM_Bv_N_per_mps*u[2]-PMLSM_Fc_N*tanh(u[2]/PMLSM_v_eps_mps))/PMLSM_M_kg
  i_alpha_calc : Fcn  Expr=u[1]*cos(u[3])-u[2]*sin(u[3])
  i_beta_calc : Fcn  Expr=u[1]*sin(u[3])+u[2]*cos(u[3])
  ib_calc : Fcn  Expr=-0.5*u[1]+sqrt(3)/2*u[2]
  ic_calc : Fcn  Expr=-0.5*u[1]-sqrt(3)/2*u[2]
  id_integrator : DiscreteIntegrator  gainval=1  SampleTime=PMLSM_Ts_s  ICPrevOutput=DiscIntNeverNeededParam  ICPrevScaledInput=DiscIntNeverNeededParam
  iq_integrator : DiscreteIntegrator  gainval=1  SampleTime=PMLSM_Ts_s  ICPrevOutput=DiscIntNeverNeededParam  ICPrevScaledInput=DiscIntNeverNeededParam
  omega_gain : Gain  Gain=2*pi/PMLSM_tau_NN_m
  static_current_step_enable : Constant  Value=MIL_StaticCurrentStepTest_Enable
  static_omega_select : Switch  Criteria=u2 > Threshold  Threshold=0.5  SaturateOnIntegerOverflow=off  InputSameDT=off
  static_theta_select : Switch  Criteria=u2 > Threshold  Threshold=0.5  SaturateOnIntegerOverflow=off  InputSameDT=off
  static_v_select : Switch  Criteria=u2 > Threshold  Threshold=0.5  SaturateOnIntegerOverflow=off  InputSameDT=off
  static_x_select : Switch  Criteria=u2 > Threshold  Threshold=0.5  SaturateOnIntegerOverflow=off  InputSameDT=off
  static_zero : Constant  Value=0
  theta_calc : Fcn  Expr=rem(2*pi*u[1]/PMLSM_tau_NN_m+PMLSM_theta_offset_rad,2*pi)
  v_integrator : DiscreteIntegrator  gainval=1  SampleTime=PMLSM_Ts_s  ICPrevOutput=DiscIntNeverNeededParam  ICPrevScaledInput=DiscIntNeverNeededParam
  v_to_mmps : Gain  Gain=1000
  x_integrator : DiscreteIntegrator  gainval=1  SampleTime=PMLSM_Ts_s  ICPrevOutput=DiscIntNeverNeededParam  ICPrevScaledInput=DiscIntNeverNeededParam
  x_to_mm : Gain  Gain=1000
  id : Outport
  iq : Outport  Port=2
  ia : Outport  Port=3
  ib : Outport  Port=4
  ic : Outport  Port=5
  x_mm : Outport  Port=6
  v_mmps : Outport  Port=7
  theta_e_actual : Outport  Port=8
  omega_e : Outport  Port=9
  wires:
  vd/1 -> did_mux/1
  id_integrator/1 -> id/1, abc_mux/1, diq_mux/4, did_mux/2
  iq_integrator/1 -> diq_mux/2, force_mux/1, did_mux/4, iq/1, abc_mux/2
  did_mux/1 -> did_dt/1
  did_dt/1 -> id_integrator/1
  vq/1 -> diq_mux/1
  diq_mux/1 -> diq_dt/1
  diq_dt/1 -> iq_integrator/1
  v_integrator/1 -> x_integrator/1, v_to_mmps/1, omega_gain/1, force_mux/2
  load_force/1 -> force_mux/3
  force_mux/1 -> force_to_dv/1
  force_to_dv/1 -> v_integrator/1
  x_integrator/1 -> theta_calc/1, x_to_mm/1
  abc_mux/1 -> i_beta_calc/1, i_alpha_calc/1
  i_alpha_calc/1 -> ia/1, alpha_beta_mux/1
  i_beta_calc/1 -> alpha_beta_mux/2
  alpha_beta_mux/1 -> ib_calc/1, ic_calc/1
  ib_calc/1 -> ib/1
  ic_calc/1 -> ic/1
  static_zero/1 -> [static_freeze_zero]
  static_current_step_enable/1 -> [static_freeze_enable]
  [static_freeze_zero] -> static_theta_select/1
  [static_freeze_enable] -> static_theta_select/2
  theta_calc/1 -> static_theta_select/3
  static_theta_select/1 -> theta_e_actual/1, [static_theta_for_abc]
  [static_theta_for_abc] -> abc_mux/3
  [static_freeze_zero] -> static_x_select/1
  [static_freeze_enable] -> static_x_select/2
  x_to_mm/1 -> static_x_select/3
  static_x_select/1 -> x_mm/1
  [static_freeze_zero] -> static_v_select/1
  [static_freeze_enable] -> static_v_select/2
  v_to_mmps/1 -> static_v_select/3
  static_v_select/1 -> v_mmps/1
  [static_freeze_zero] -> static_omega_select/1
  [static_freeze_enable] -> static_omega_select/2
  omega_gain/1 -> static_omega_select/3
  static_omega_select/1 -> omega_e/1, [static_omega_for_elec]
  [static_omega_for_elec] -> did_mux/3
  [static_omega_for_elec] -> diq_mux/3

== system PMLSM_MIL_ControlCore_Sim/Power_Plant_Feedback/Sensor_Model ==
  ia : Inport
  ib : Inport  Port=2
  ic : Inport  Port=3
  x_mm : Inport  Port=4
  diff_to_speed : Gain  Gain=1/(PMLSM_sensor_delay_samples*PMLSM_Ts_s)
  x_delay_50 : Delay  DelayLength=PMLSM_sensor_delay_samples  InitialCondition=0  SampleTime=PMLSM_Ts_s
  x_diff : Sum  Inputs=+-
  x_quant_1um : Fcn  Expr=floor(u[1]/PMLSM_grating_resolution_mm+0.5)*PMLSM_grating_resolution_mm
  ia_meas : Outport
  ib_meas : Outport  Port=2
  ic_meas : Outport  Port=3
  x_meas_mm : Outport  Port=4
  v_meas_mmps : Outport  Port=5
  wires:
  diff_to_speed/1 -> v_meas_mmps/1
  ib/1 -> ib_meas/1
  ia/1 -> ia_meas/1
  x_diff/1 -> diff_to_speed/1
  x_delay_50/1 -> x_diff/2
  x_quant_1um/1 -> x_delay_50/1, x_diff/1, x_meas_mm/1
  x_mm/1 -> x_quant_1um/1
  ic/1 -> ic_meas/1

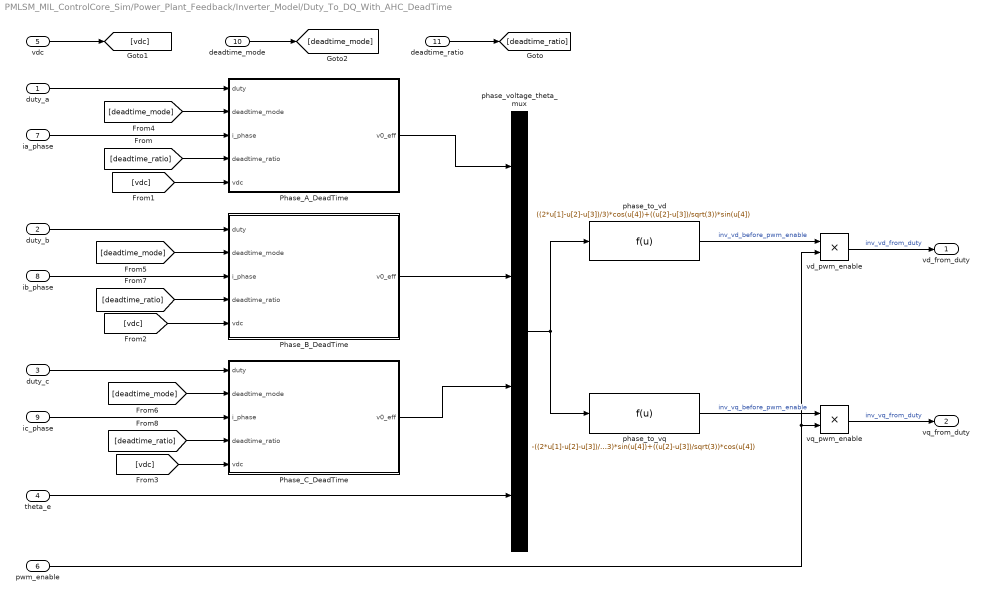
== system PMLSM_MIL_ControlCore_Sim/Power_Plant_Feedback/Inverter_Model/Duty_To_DQ_With_AHC_DeadTime ==
  duty_a : Inport
  duty_b : Inport  Port=2
  duty_c : Inport  Port=3
  theta_e : Inport  Port=4
  vdc : Inport  Port=5
  pwm_enable : Inport  Port=6
  ia_phase : Inport  Port=7
  ib_phase : Inport  Port=8
  ic_phase : Inport  Port=9
  deadtime_mode : Inport  Port=10
  deadtime_ratio : Inport  Port=11
  Phase_A_DeadTime : Subsystem
  Phase_B_DeadTime : Subsystem
  Phase_C_DeadTime : Subsystem
  phase_to_vd : Fcn  Expr=((2*u[1]-u[2]-u[3])/3)*cos(u[4])+((u[2]-u[3])/sqrt(3))*sin(u[4])
  phase_to_vq : Fcn  Expr=-((2*u[1]-u[2]-u[3])/3)*sin(u[4])+((u[2]-u[3])/sqrt(3))*cos(u[4])
  phase_voltage_theta_mux : Mux
  vd_pwm_enable : Product
  vq_pwm_enable : Product
  vd_from_duty : Outport
  vq_from_duty : Outport  Port=2
  wires:
  duty_a/1 -> Phase_A_DeadTime/1(duty)
  ia_phase/1 -> Phase_A_DeadTime/3(i_phase)
  duty_b/1 -> Phase_B_DeadTime/1(duty)
  ib_phase/1 -> Phase_B_DeadTime/3(i_phase)
  duty_c/1 -> Phase_C_DeadTime/1(duty)
  ic_phase/1 -> Phase_C_DeadTime/3(i_phase)
  Phase_A_DeadTime/1(v0_eff) -> phase_voltage_theta_mux/1
  Phase_B_DeadTime/1(v0_eff) -> phase_voltage_theta_mux/2
  Phase_C_DeadTime/1(v0_eff) -> phase_voltage_theta_mux/3
  theta_e/1 -> phase_voltage_theta_mux/4
  phase_voltage_theta_mux/1 -> phase_to_vq/1, phase_to_vd/1
  phase_to_vd/1 -> vd_pwm_enable/1  "inv_vd_before_pwm_enable"
  pwm_enable/1 -> vd_pwm_enable/2, vq_pwm_enable/2
  phase_to_vq/1 -> vq_pwm_enable/1  "inv_vq_before_pwm_enable"
  vd_pwm_enable/1 -> vd_from_duty/1  "inv_vd_from_duty"
  vq_pwm_enable/1 -> vq_from_duty/1  "inv_vq_from_duty"
  deadtime_ratio/1 -> [deadtime_ratio]
  vdc/1 -> [vdc]
  [vdc] -> Phase_A_DeadTime/5(vdc)
  [vdc] -> Phase_B_DeadTime/5(vdc)
  [vdc] -> Phase_C_DeadTime/5(vdc)
  deadtime_mode/1 -> [deadtime_mode]
  [deadtime_mode] -> Phase_A_DeadTime/2(deadtime_mode)
  [deadtime_mode] -> Phase_B_DeadTime/2(deadtime_mode)
  [deadtime_mode] -> Phase_C_DeadTime/2(deadtime_mode)
  [deadtime_ratio] -> Phase_A_DeadTime/4(deadtime_ratio)
  [deadtime_ratio] -> Phase_B_DeadTime/4(deadtime_ratio)
  [deadtime_ratio] -> Phase_C_DeadTime/4(deadtime_ratio)

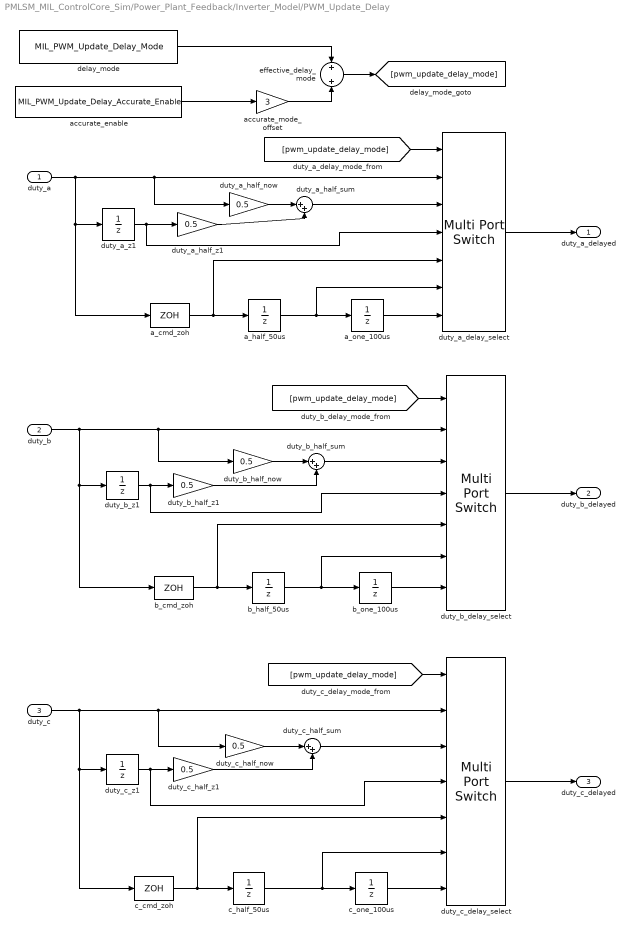
== system PMLSM_MIL_ControlCore_Sim/Power_Plant_Feedback/Inverter_Model/PWM_Update_Delay ==
  duty_a : Inport
  duty_b : Inport  Port=2
  duty_c : Inport  Port=3
  a_cmd_zoh : ZeroOrderHold  SampleTime=MIL_Current_Control_Ts_s
  a_half_50us : UnitDelay  InitialCondition=0.5  SampleTime=MIL_PWM_Delay_Substep_s
  a_one_100us : UnitDelay  InitialCondition=0.5  SampleTime=MIL_PWM_Delay_Substep_s
  accurate_enable : Constant  Value=MIL_PWM_Update_Delay_Accurate_Enable
  accurate_mode_offset : Gain  Gain=3
  b_cmd_zoh : ZeroOrderHold  SampleTime=MIL_Current_Control_Ts_s
  b_half_50us : UnitDelay  InitialCondition=0.5  SampleTime=MIL_PWM_Delay_Substep_s
  b_one_100us : UnitDelay  InitialCondition=0.5  SampleTime=MIL_PWM_Delay_Substep_s
  c_cmd_zoh : ZeroOrderHold  SampleTime=MIL_Current_Control_Ts_s
  c_half_50us : UnitDelay  InitialCondition=0.5  SampleTime=MIL_PWM_Delay_Substep_s
  c_one_100us : UnitDelay  InitialCondition=0.5  SampleTime=MIL_PWM_Delay_Substep_s
  delay_mode : Constant  Value=MIL_PWM_Update_Delay_Mode
  duty_a_delay_select : MultiPortSwitch  DataPortOrder=Zero-based contiguous  Inputs=6  zeroidx=on  SaturateOnIntegerOverflow=off  InputSameDT=off
  duty_a_half_now : Gain  Gain=0.5
  duty_a_half_sum : Sum  Inputs=|++
  duty_a_half_z1 : Gain  Gain=0.5
  duty_a_z1 : UnitDelay  InitialCondition=0.5  SampleTime=Ts_ACR
  duty_b_delay_select : MultiPortSwitch  DataPortOrder=Zero-based contiguous  Inputs=6  zeroidx=on  SaturateOnIntegerOverflow=off  InputSameDT=off
  duty_b_half_now : Gain  Gain=0.5
  duty_b_half_sum : Sum  Inputs=|++
  duty_b_half_z1 : Gain  Gain=0.5
  duty_b_z1 : UnitDelay  InitialCondition=0.5  SampleTime=Ts_ACR
  duty_c_delay_select : MultiPortSwitch  DataPortOrder=Zero-based contiguous  Inputs=6  zeroidx=on  SaturateOnIntegerOverflow=off  InputSameDT=off
  duty_c_half_now : Gain  Gain=0.5
  duty_c_half_sum : Sum  Inputs=|++
  duty_c_half_z1 : Gain  Gain=0.5
  duty_c_z1 : UnitDelay  InitialCondition=0.5  SampleTime=Ts_ACR
  effective_delay_mode : Sum
  duty_a_delayed : Outport
  duty_b_delayed : Outport  Port=2
  duty_c_delayed : Outport  Port=3
  wires:
  duty_a/1 -> a_cmd_zoh/1, duty_a_z1/1, duty_a_half_now/1, duty_a_delay_select/2
  duty_a_z1/1 -> duty_a_delay_select/4, duty_a_half_z1/1
  duty_a_half_now/1 -> duty_a_half_sum/1
  duty_a_half_z1/1 -> duty_a_half_sum/2
  [pwm_update_delay_mode] -> duty_a_delay_select/1
  duty_a_half_sum/1 -> duty_a_delay_select/3
  duty_a_delay_select/1 -> duty_a_delayed/1
  duty_b/1 -> b_cmd_zoh/1, duty_b_z1/1, duty_b_half_now/1, duty_b_delay_select/2
  duty_b_z1/1 -> duty_b_delay_select/4, duty_b_half_z1/1
  duty_b_half_now/1 -> duty_b_half_sum/1
  duty_b_half_z1/1 -> duty_b_half_sum/2
  [pwm_update_delay_mode] -> duty_b_delay_select/1
  duty_b_half_sum/1 -> duty_b_delay_select/3
  duty_b_delay_select/1 -> duty_b_delayed/1
  duty_c/1 -> c_cmd_zoh/1, duty_c_z1/1, duty_c_half_now/1, duty_c_delay_select/2
  duty_c_z1/1 -> duty_c_delay_select/4, duty_c_half_z1/1
  duty_c_half_now/1 -> duty_c_half_sum/1
  duty_c_half_z1/1 -> duty_c_half_sum/2
  [pwm_update_delay_mode] -> duty_c_delay_select/1
  duty_c_half_sum/1 -> duty_c_delay_select/3
  duty_c_delay_select/1 -> duty_c_delayed/1
  accurate_enable/1 -> accurate_mode_offset/1
  delay_mode/1 -> effective_delay_mode/1
  accurate_mode_offset/1 -> effective_delay_mode/2
  effective_delay_mode/1 -> [pwm_update_delay_mode]
  a_cmd_zoh/1 -> duty_a_delay_select/5, a_half_50us/1
  a_half_50us/1 -> duty_a_delay_select/6, a_one_100us/1
  a_one_100us/1 -> duty_a_delay_select/7
  b_cmd_zoh/1 -> duty_b_delay_select/5, b_half_50us/1
  b_half_50us/1 -> duty_b_delay_select/6, b_one_100us/1
  b_one_100us/1 -> duty_b_delay_select/7
  c_cmd_zoh/1 -> duty_c_delay_select/5, c_half_50us/1
  c_half_50us/1 -> duty_c_delay_select/6, c_one_100us/1
  c_one_100us/1 -> duty_c_delay_select/7

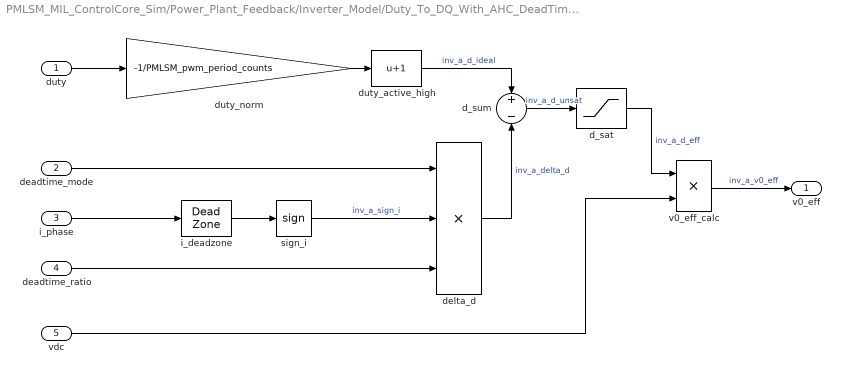
== system PMLSM_MIL_ControlCore_Sim/Power_Plant_Feedback/Inverter_Model/Duty_To_DQ_With_AHC_DeadTime/Phase_A_DeadTime ==
  duty : Inport
  deadtime_mode : Inport  Port=2
  i_phase : Inport  Port=3
  deadtime_ratio : Inport  Port=4
  vdc : Inport  Port=5
  d_sat : Saturate  UpperLimit=1  LowerLimit=0
  d_sum : Sum  Inputs=+-
  delta_d : Product  Inputs=3
  duty_active_high : Bias  Bias=1  SaturateOnIntegerOverflow=off
  duty_norm : Gain  Gain=-1/PMLSM_pwm_period_counts
  i_deadzone : DeadZone  LowerValue=-PMLSM_deadtime_current_eps_A  UpperValue=PMLSM_deadtime_current_eps_A
  sign_i : Signum
  v0_eff_calc : Product
  v0_eff : Outport
  wires:
  duty/1 -> duty_norm/1
  duty_norm/1 -> duty_active_high/1
  duty_active_high/1 -> d_sum/1  "inv_a_d_ideal"
  i_phase/1 -> i_deadzone/1
  i_deadzone/1 -> sign_i/1
  deadtime_mode/1 -> delta_d/1
  sign_i/1 -> delta_d/2  "inv_a_sign_i"
  deadtime_ratio/1 -> delta_d/3
  delta_d/1 -> d_sum/2  "inv_a_delta_d"
  d_sum/1 -> d_sat/1  "inv_a_d_unsat"
  d_sat/1 -> v0_eff_calc/1  "inv_a_d_eff"
  vdc/1 -> v0_eff_calc/2
  v0_eff_calc/1 -> v0_eff/1  "inv_a_v0_eff"

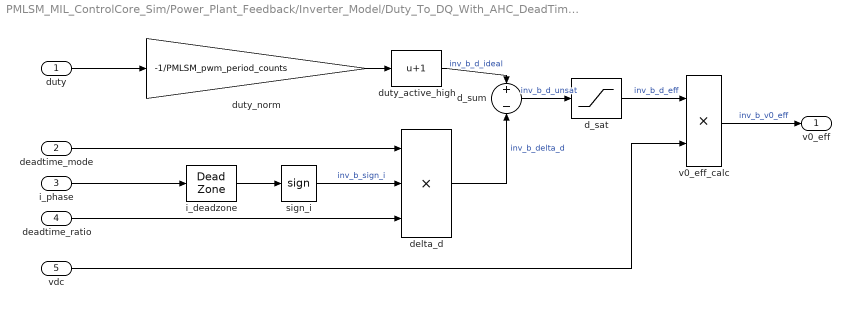
== system PMLSM_MIL_ControlCore_Sim/Power_Plant_Feedback/Inverter_Model/Duty_To_DQ_With_AHC_DeadTime/Phase_B_DeadTime ==
  duty : Inport
  deadtime_mode : Inport  Port=2
  i_phase : Inport  Port=3
  deadtime_ratio : Inport  Port=4
  vdc : Inport  Port=5
  d_sat : Saturate  UpperLimit=1  LowerLimit=0
  d_sum : Sum  Inputs=+-
  delta_d : Product  Inputs=3
  duty_active_high : Bias  Bias=1  SaturateOnIntegerOverflow=off
  duty_norm : Gain  Gain=-1/PMLSM_pwm_period_counts
  i_deadzone : DeadZone  LowerValue=-PMLSM_deadtime_current_eps_A  UpperValue=PMLSM_deadtime_current_eps_A
  sign_i : Signum
  v0_eff_calc : Product
  v0_eff : Outport
  wires:
  duty/1 -> duty_norm/1
  duty_norm/1 -> duty_active_high/1
  duty_active_high/1 -> d_sum/1  "inv_b_d_ideal"
  i_phase/1 -> i_deadzone/1
  i_deadzone/1 -> sign_i/1
  deadtime_mode/1 -> delta_d/1
  sign_i/1 -> delta_d/2  "inv_b_sign_i"
  deadtime_ratio/1 -> delta_d/3
  delta_d/1 -> d_sum/2  "inv_b_delta_d"
  d_sum/1 -> d_sat/1  "inv_b_d_unsat"
  d_sat/1 -> v0_eff_calc/1  "inv_b_d_eff"
  vdc/1 -> v0_eff_calc/2
  v0_eff_calc/1 -> v0_eff/1  "inv_b_v0_eff"

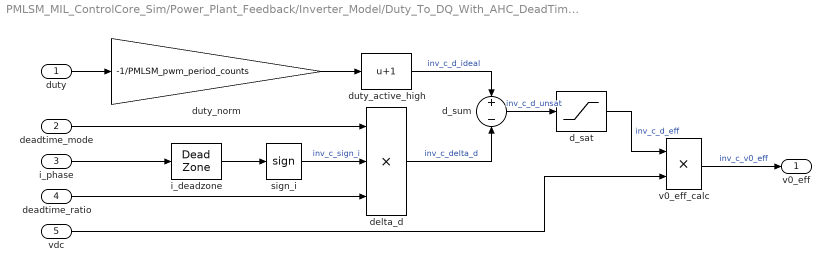
== system PMLSM_MIL_ControlCore_Sim/Power_Plant_Feedback/Inverter_Model/Duty_To_DQ_With_AHC_DeadTime/Phase_C_DeadTime ==
  duty : Inport
  deadtime_mode : Inport  Port=2
  i_phase : Inport  Port=3
  deadtime_ratio : Inport  Port=4
  vdc : Inport  Port=5
  d_sat : Saturate  UpperLimit=1  LowerLimit=0
  d_sum : Sum  Inputs=+-
  delta_d : Product  Inputs=3
  duty_active_high : Bias  Bias=1  SaturateOnIntegerOverflow=off
  duty_norm : Gain  Gain=-1/PMLSM_pwm_period_counts
  i_deadzone : DeadZone  LowerValue=-PMLSM_deadtime_current_eps_A  UpperValue=PMLSM_deadtime_current_eps_A
  sign_i : Signum
  v0_eff_calc : Product
  v0_eff : Outport
  wires:
  duty/1 -> duty_norm/1
  duty_norm/1 -> duty_active_high/1
  duty_active_high/1 -> d_sum/1  "inv_c_d_ideal"
  i_phase/1 -> i_deadzone/1
  i_deadzone/1 -> sign_i/1
  deadtime_mode/1 -> delta_d/1
  sign_i/1 -> delta_d/2  "inv_c_sign_i"
  deadtime_ratio/1 -> delta_d/3
  delta_d/1 -> d_sum/2  "inv_c_delta_d"
  d_sum/1 -> d_sat/1  "inv_c_d_unsat"
  d_sat/1 -> v0_eff_calc/1  "inv_c_d_eff"
  vdc/1 -> v0_eff_calc/2
  v0_eff_calc/1 -> v0_eff/1  "inv_c_v0_eff"

== matlab function PMLSM_MIL_ControlCore_Sim/Startup_And_Commands/Startup_Enable_Sequencer ==
  data: t input size=1; enable_cmd output size=1; init_done input size=1; MIL_Mode input size=1; fault_i output size=1; fault_u output size=1; close_loop_en output size=1; init_start output size=1; init_reset output size=1; pi_reset_en output size=1; pwm_enable output size=1; MIL_Ts_s parameter; MIL_EnableTime_s parameter; MIL_InitDoneDelay_s parameter; MIL_Fault_Test_Case parameter; MIL_Fault_Start_s parameter
function [enable_cmd,fault_i,fault_u,close_loop_en,init_start,init_reset,pi_reset_en,pwm_enable] = fcn(t, init_done, MIL_Mode, MIL_Ts_s, MIL_EnableTime_s, MIL_InitDoneDelay_s, MIL_Fault_Test_Case, MIL_Fault_Start_s)
%#codegen
persistent init_done_timer_s
if isempty(init_done_timer_s)
    init_done_timer_s = 0;
end
enable_cmd = 0;
fault_i = 0;
fault_u = 0;
close_loop_en = 0;
init_start = 0;
init_reset = 1;
pi_reset_en = 1;
pwm_enable = 0;
if t >= MIL_EnableTime_s
    enable_cmd = 1;
    init_start = 1;
    init_reset = 0;
    pi_reset_en = 0;
end
if MIL_Fault_Test_Case == 1 && t >= MIL_Fault_Start_s
    fault_i = 1;
elseif MIL_Fault_Test_Case == 2 && t >= MIL_Fault_Start_s
    fault_u = 1;
elseif MIL_Fault_Test_Case == 3 && t >= MIL_Fault_Start_s
    enable_cmd = 0;
end
if enable_cmd ~= 0 && init_done ~= 0 && fault_i == 0 && fault_u == 0
    init_done_timer_s = init_done_timer_s + MIL_Ts_s;
else
    init_done_timer_s = 0;
end
if enable_cmd ~= 0 && MIL_Mode ~= 1 && init_done_timer_s >= MIL_InitDoneDelay_s
    close_loop_en = 1;
end
if enable_cmd ~= 0 && fault_i == 0 && fault_u == 0
    pwm_enable = 1;
else
    pwm_enable = 0;
end
end

== matlab function PMLSM_MIL_ControlCore_Sim/Startup_And_Commands/Simple_Command_Profile ==
  data: t input size=1; iq_test_mode output size=1; init_done input size=1; close_loop_en input size=1; MIL_Mode input size=1; iq_test_ref output size=1; v_ref_cmd_mmps output size=1; x_ref_mm output size=1; load_force output size=1; vdc output size=1; pos_loop_en output size=1; id_ref_set output size=1; x_override_enable output size=1; x_override_mm output size=1; MIL_Ts_s parameter; MIL_SpeedCommand_mmps parameter; MIL_PositiveSpeedDuration_s parameter; MIL_ZeroSpeedDuration_s parameter; MIL_NegativeSpeedDuration_s parameter; MIL_IqInjection_A parameter; MIL_IqInjectionDelay_s parameter; MIL_IqRefRampTime_s parameter; MIL_IqPositiveDuration_s parameter; MIL_IqZeroDuration_s parameter; MIL_IqNegativeDuration_s parameter; MIL_IqCycleCount parameter; MIL_PositionStep_mm parameter; MIL_PositionStepDelay_s parameter; MIL_LoadForce_N parameter; MIL_Vdc_V parameter; MIL_LoadStartRel_s parameter; MIL_LoadEndRel_s parameter
function [iq_test_mode,iq_test_ref,v_ref_cmd_mmps,x_ref_mm,load_force,vdc,pos_loop_en,id_ref_set,x_override_enable,x_override_mm] = fcn(t, init_done, close_loop_en, MIL_Mode, MIL_Ts_s, MIL_SpeedCommand_mmps, MIL_PositiveSpeedDuration_s, MIL_ZeroSpeedDuration_s, MIL_NegativeSpeedDuration_s, MIL_IqInjection_A, MIL_IqInjectionDelay_s, MIL_IqRefRampTime_s, MIL_IqPositiveDuration_s, MIL_IqZeroDuration_s, MIL_IqNegativeDuration_s, MIL_IqCycleCount, MIL_PositionStep_mm, MIL_PositionStepDelay_s, MIL_LoadForce_N, MIL_Vdc_V, MIL_LoadStartRel_s, MIL_LoadEndRel_s)
%#codegen
persistent test_timer_s
if isempty(test_timer_s)
    test_timer_s = 0;
end
iq_test_mode = 0;
iq_test_ref = 0;
v_ref_cmd_mmps = 0;
x_ref_mm = 0;
load_force = 0;
vdc = MIL_Vdc_V;
pos_loop_en = 0;
id_ref_set = 0;
x_override_enable = 0;
x_override_mm = 0;
if (MIL_Mode == 1 && init_done ~= 0) || (MIL_Mode == 4 && init_done ~= 0 && close_loop_en ~= 0) || (MIL_Mode ~= 1 && MIL_Mode ~= 4 && init_done ~= 0 && close_loop_en ~= 0)
    test_timer_s = test_timer_s + MIL_Ts_s;
else
    test_timer_s = 0;
end
if init_done ~= 0 && close_loop_en ~= 0 && ...
        test_timer_s >= MIL_LoadStartRel_s && ...
        test_timer_s < MIL_LoadEndRel_s
    load_force = MIL_LoadForce_N;
end
switch MIL_Mode
    case {1, 4}
        if init_done == 0
            return;
        end
        cycle_period_s = MIL_IqPositiveDuration_s + MIL_IqZeroDuration_s + MIL_IqNegativeDuration_s + MIL_IqZeroDuration_s;
        cycle_time_s = test_timer_s - MIL_IqInjectionDelay_s;
        if cycle_time_s < 0 || cycle_period_s <= 0
            return;
        end
        cycle_index = floor(cycle_time_s / cycle_period_s);
        phase_s = cycle_time_s - cycle_index * cycle_period_s;
        if cycle_index >= MIL_IqCycleCount
            return;
        end
        iq_test_mode = 1;
        ramp_s = MIL_IqRefRampTime_s;
        pos_ramp_s = min(ramp_s, 0.5*MIL_IqPositiveDuration_s);
        neg_ramp_s = min(ramp_s, 0.5*MIL_IqNegativeDuration_s);
        pos_end_s = MIL_IqPositiveDuration_s;
        neg_start_s = MIL_IqPositiveDuration_s + MIL_IqZeroDuration_s;
        neg_end_s = neg_start_s + MIL_IqNegativeDuration_s;
        if phase_s < pos_end_s
            if pos_ramp_s > 0 && phase_s < pos_ramp_s
                iq_test_ref = MIL_IqInjection_A * phase_s / pos_ramp_s;
            elseif pos_ramp_s > 0 && phase_s > pos_end_s - pos_ramp_s
                iq_test_ref = MIL_IqInjection_A * (pos_end_s - phase_s) / pos_ramp_s;
            else
                iq_test_ref = MIL_IqInjection_A;
            end
        elseif phase_s >= neg_start_s && phase_s < neg_end_s
            if neg_ramp_s > 0 && phase_s < neg_start_s + neg_ramp_s
                iq_test_ref = -MIL_IqInjection_A * (phase_s - neg_start_s) / neg_ramp_s;
            elseif neg_ramp_s > 0 && phase_s > neg_end_s - neg_ramp_s
                iq_test_ref = -MIL_IqInjection_A * (neg_end_s - phase_s) / neg_ramp_s;
            else
                iq_test_ref = -MIL_IqInjection_A;
            end
        end
    case 2
        if init_done == 0 || close_loop_en == 0
            return;
        end
        t1 = MIL_PositiveSpeedDuration_s;
        t2 = MIL_PositiveSpeedDuration_s + MIL_ZeroSpeedDuration_s;
        t3 = MIL_PositiveSpeedDuration_s + MIL_ZeroSpeedDuration_s + MIL_NegativeSpeedDuration_s;
        if test_timer_s < t1
            v_ref_cmd_mmps = MIL_SpeedCommand_mmps;
        elseif test_timer_s < t2
            v_ref_cmd_mmps = 0;
        elseif test_timer_s < t3
            v_ref_cmd_mmps = -MIL_SpeedCommand_mmps;
        else
            v_ref_cmd_mmps = 0;
        end
    case 3
        if init_done == 0 || close_loop_en == 0
            return;
        end
        pos_loop_en = 1;
        if test_timer_s >= MIL_PositionStepDelay_s
            x_ref_mm = MIL_PositionStep_mm;
        end
end
